simulink model "Robot_Unicycle"  (R2024b)
settings: Solver=FixedStepAuto  StartTime=0.0  StopTime=100  FixedStep=0.01  RelTol=1e-3
libraries: fuzblock x1
settings Model: Creator=azonh  LastModifiedBy=azonh

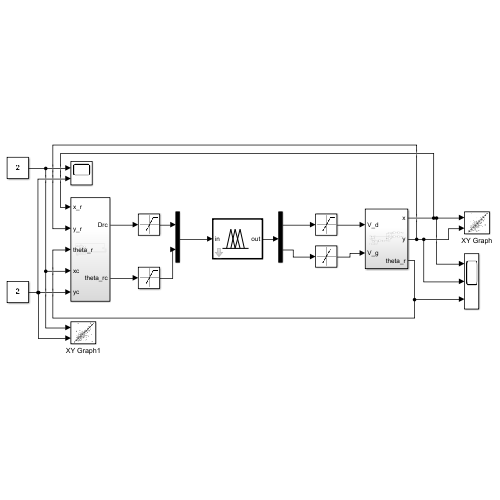
[thumbnail: Simulink's stored preview of the top-level diagram]
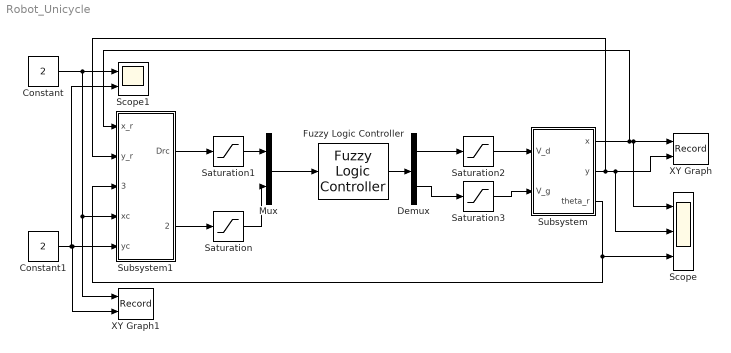
== system Robot_Unicycle ==
  Constant : Constant  Value=2
  Constant1 : Constant  Value=2
  Demux : Demux  Outputs=2
  Fuzzy Logic Controller : fuzblock/Fuzzy Logic  Controller  FIS='Controller_fuzzy.fis'  OutputSampleNumber=101  DataType=double  FuzzifiedInputs=off  RuleFiringStrengths=off  RuleOutputs=off  AggregatedOutputs=off  SimulateUsing=Interpreted execution  OutOfRangeInputValueMessage=warning  NoRuleFiredMessage=warning  EmptyOutputFuzzySetMessage=warning
  Mux : Mux  Inputs=2
  Saturation : Saturate  UpperLimit=pi  LowerLimit=-pi
  Saturation1 : Saturate  UpperLimit=2  LowerLimit=0
  Saturation2 : Saturate  LowerLimit=0
  Saturation3 : Saturate  LowerLimit=0
  Scope : Scope  NumInputPorts=3
  Scope1 : Scope  NumInputPorts=2
  Subsystem : Subsystem
  Subsystem1 : Subsystem
  XY Graph : Record  FileSettingsInternal="{\"entries\":[{\"content\":{\"excelSettings\":{\"content\":{},\"type\":\"Streamout.ExcelSettings\"}},\"type\":\"Streamout.FileSettingStorage\",\"uuid\":\"\"}],\"packageUris\":[\"http:\\/\\/schema.mathworks.com\\/mf0\\/streamout_blocks\\/R2020a\"],\"version\":\"1.0\"}"  Layout=[1 1]  SignalsInternal="{\"entries\":[{\"content\":{\"signals\":[{\"content\":{\"blockPath\":[],\"dimensions\":[1],\"domain\":\"\",\"lineColor\":\"#a2142f\",\"plots\":[ 1 ],\"port\":1,\"sid\":[\"\"],\"signalID\":1,\"signalName\":\"Subsystem:1\"},\"type\":\"RecordBlkView.Signal\",\"uuid\":\"\"},{\"content\":{\"blockPath\":[],\"dimensions\":[1],\"domain\":\"\",\"lineColor\":\"#139fff\",\"plots\":[ 1 ],\"port\":2,\"sid\":[\"\"],\"signalID\":2,\"signalName\":\"Subsystem:2\"},\"type\":\"RecordBlkView.Signal\",\"uuid\":\"\"}]},\"type\":\"RecordBlkView.InputSignals\",\"uuid\":\"\"}],\"packageUris\":[\"http:\\/\\/schema.mathworks.com\\/mf0\\/streamout_blocks\\/R2020a\"],\"version\":\"1.0\"}"  VisualizationBindings="{\"xyplotplugin\":{\"info\":[{\"series\":[{\"bindingParametersList\":[{\"parameter\":\"X-Axis\",\"signalID\":1,\"signalName\":\"Subsystem:1\"},{\"parameter\":\"Y-Axis\",\"signalID\":2,\"signalName\":\"Subsystem:2\"}],\"seriesID\":0}],\"subplotID\":1}]}}"  CompatibilityTag=XY
  XY Graph1 : Record  FileSettingsInternal="{\"entries\":[{\"content\":{\"excelSettings\":{\"content\":{},\"type\":\"Streamout.ExcelSettings\"}},\"type\":\"Streamout.FileSettingStorage\",\"uuid\":\"\"}],\"packageUris\":[\"http:\\/\\/schema.mathworks.com\\/mf0\\/streamout_blocks\\/R2020a\"],\"version\":\"1.0\"}"  Layout=[1 1]  SignalsInternal="{\"entries\":[{\"content\":{\"signals\":[{\"content\":{\"blockPath\":[],\"dimensions\":[1],\"domain\":\"\",\"lineColor\":\"#a2142f\",\"plots\":[ 1 ],\"port\":1,\"sid\":[\"\"],\"signalID\":1,\"signalName\":\"Constant\"},\"type\":\"RecordBlkView.Signal\",\"uuid\":\"\"},{\"content\":{\"blockPath\":[],\"dimensions\":[1],\"domain\":\"\",\"lineColor\":\"#139fff\",\"plots\":[ 1 ],\"port\":2,\"sid\":[\"\"],\"signalID\":2,\"signalName\":\"Constant1\"},\"type\":\"RecordBlkView.Signal\",\"uuid\":\"\"}]},\"type\":\"RecordBlkView.InputSignals\",\"uuid\":\"\"}],\"packageUris\":[\"http:\\/\\/schema.mathworks.com\\/mf0\\/streamout_blocks\\/R2020a\"],\"version\":\"1.0\"}"  VisualizationBindings="{\"xyplotplugin\":{\"info\":[{\"series\":[{\"bindingParametersList\":[{\"parameter\":\"X-Axis\",\"signalID\":1,\"signalName\":\"Constant\"},{\"parameter\":\"Y-Axis\",\"signalID\":2,\"signalName\":\"Constant1\"}],\"seriesID\":0}],\"subplotID\":1}]}}"  CompatibilityTag=XY
  wires:
  Constant1/1 -> Subsystem1/5(yc), XY Graph1/2, Scope1/2
  Constant/1 -> XY Graph1/1, Subsystem1/4(xc), Scope1/1
  Saturation1/1 -> Mux/1
  Subsystem1/2(theta_rc) -> Saturation/1
  Subsystem1/1(Drc) -> Saturation1/1
  Demux/1 -> Saturation2/1
  Fuzzy Logic Controller/1 -> Demux/1
  Mux/1 -> Fuzzy Logic Controller/1
  Saturation/1 -> Mux/2
  Demux/2 -> Saturation3/1
  Saturation2/1 -> Subsystem/1(V_d)
  Saturation3/1 -> Subsystem/2(V_g)
  Subsystem/1(x) -> Scope/1, XY Graph/1, Subsystem1/1(x_r)
  Subsystem/2(y) -> Scope/2, XY Graph/2, Subsystem1/2(y_r)
  Subsystem/3(theta_r) -> Subsystem1/3(theta_r), Scope/3

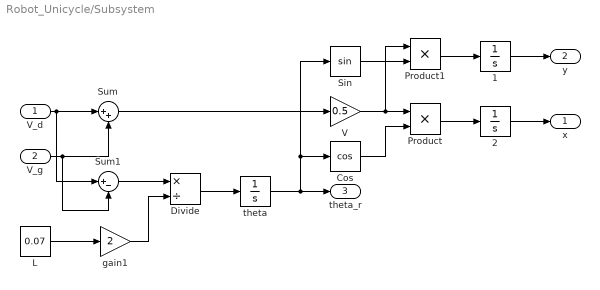
== system Robot_Unicycle/Subsystem ==
  V_d : Inport
  V_g : Inport  Port=2
  1 : Integrator
  2 : Integrator
  Cos : Trigonometry  Operator=cos
  Divide : Product  Inputs=*/
  L : Constant  Value=0.07
  Product : Product
  Product1 : Product
  Sin : Trigonometry
  Sum : Sum  Inputs=|++
  Sum1 : Sum  Inputs=|+-
  V : Gain  Gain=0.5
  gain1 : Gain  Gain=2
  theta : Integrator  InitialCondition=1  ContinuousStateAttributes='pos'
  x : Outport
  y : Outport  Port=2
  theta_r : Outport  Port=3
  wires:
  V_d/1 -> Sum1/1, Sum/1
  V_g/1 -> Sum/2, Sum1/2
  Cos/1 -> Product/2
  Divide/1 -> theta/1
  Product/1 -> 2/1
  L/1 -> gain1/1
  Sin/1 -> Product1/2
  Sum/1 -> V/1
  Sum1/1 -> Divide/1
  theta/1 -> Cos/1, Sin/1, theta_r/1
  gain1/1 -> Divide/2
  V/1 -> Product1/1, Product/1
  Product1/1 -> 1/1
  1/1 -> y/1
  2/1 -> x/1

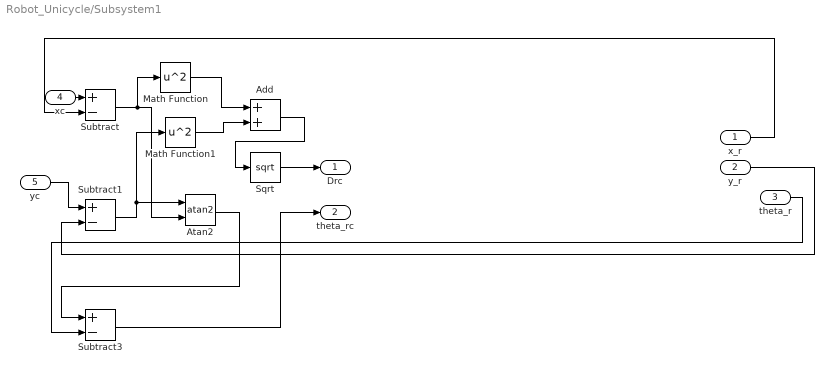
== system Robot_Unicycle/Subsystem1 ==
  x_r : Inport
  y_r : Inport  Port=2
  theta_r : Inport  Port=3
  xc : Inport  Port=4
  yc : Inport  Port=5
  Add : Sum
  Atan2 : Trigonometry  Operator=atan2
  Math Function : Math  Operator=square
  Math Function1 : Math  Operator=square
  Sqrt : Sqrt
  Subtract : Sum  Inputs=+-
  Subtract1 : Sum  Inputs=+-
  Subtract3 : Sum  Inputs=+-
  Drc : Outport
  theta_rc : Outport  Port=2
  wires:
  y_r/1 -> Subtract1/2
  Atan2/1 -> Subtract3/1
  Math Function/1 -> Add/1
  Subtract1/1 -> Atan2/1, Math Function1/1
  Subtract/1 -> Atan2/2, Math Function/1
  Math Function1/1 -> Add/2
  Add/1 -> Sqrt/1
  Subtract3/1 -> theta_rc/1
  theta_r/1 -> Subtract3/2
  x_r/1 -> Subtract/2
  Sqrt/1 -> Drc/1
  yc/1 -> Subtract1/1
  xc/1 -> Subtract/1
